simulink model "nonlinearpartd"  (R2017a)
settings: Solver=VariableStepAuto  StartTime=0.0  StopTime=3000  RelTol=1e-3
values from neighbouring files (symbols this model uses):
  g = 9.8    [CodeControlProject2.m]    (also in linear_system.m = 9.81; main.m; nonlinear_system.m = 9.81)
  Kc = lqr(A,B,Q,R)    [CodeControlProject2.m]
  l1 = 20    [CodeControlProject2.m]
  l2 = 10    [CodeControlProject2.m]
  M = 1000    [CodeControlProject2.m]    (also in main.m)
  m1 = 100    [CodeControlProject2.m]
  m2 = 100    [CodeControlProject2.m]
settings Model: Creator=Parth Jindal  LastModifiedBy=Parth Jindal

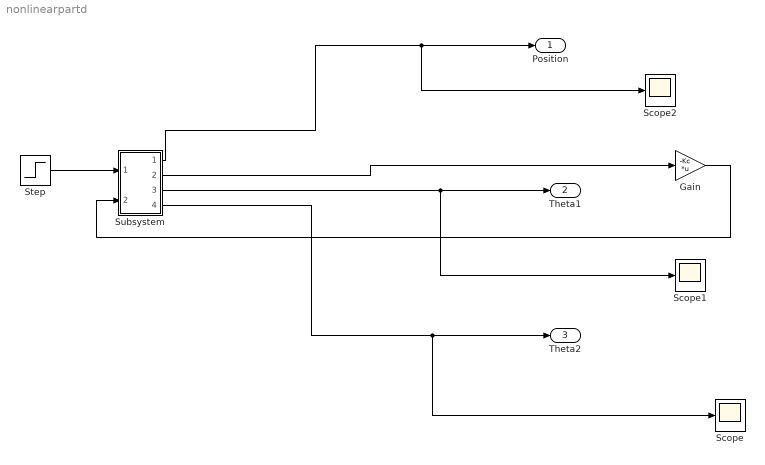
== system nonlinearpartd ==
  Gain : Gain  Gain=-Kc  Multiplication=Matrix(K*u)
  Scope : Scope
  Scope1 : Scope
  Scope2 : Scope
  Step : Step  SampleTime=0
  Subsystem : Subsystem
  Position : Outport
  Theta1 : Outport  Port=2
  Theta2 : Outport  Port=3
  wires:
  Subsystem/3(Out3) -> Scope1/1, Theta1/1
  Subsystem/4(Out4) -> Scope/1, Theta2/1
  Gain/1 -> Subsystem/2(In2)
  Subsystem/2(Out2) -> Gain/1
  Step/1 -> Subsystem/1(In1)
  Subsystem/1(Out1) -> Scope2/1, Position/1

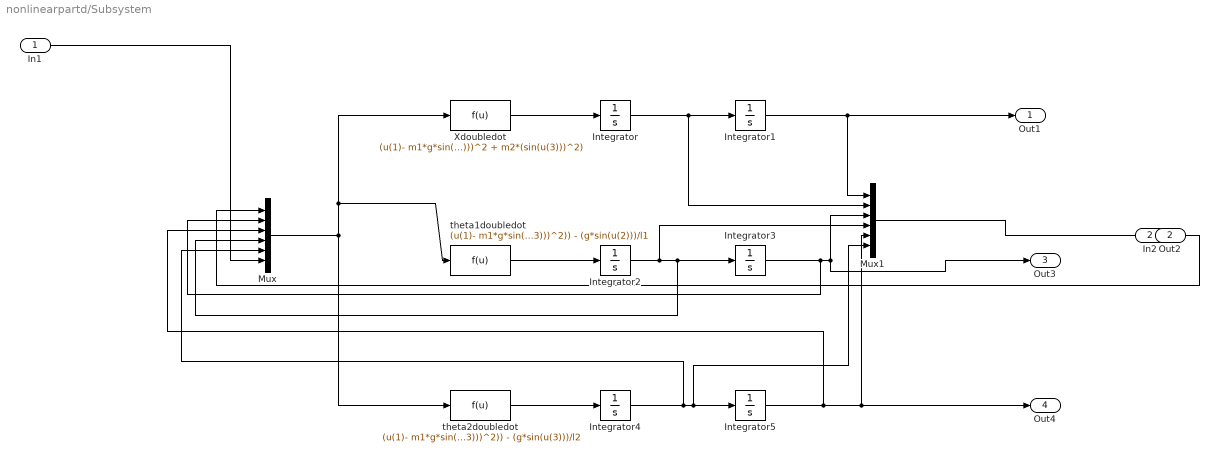
== system nonlinearpartd/Subsystem ==
  In1 : Inport
  In2 : Inport  Port=2
  Integrator{,2..5} (5 alike) : Integrator
  Integrator1 : Integrator  InitialCondition=-4
  Mux : Mux  Inputs=6
  Mux1 : Mux  Inputs=6
  Xdoubledot : Fcn  Expr=(u(1)- m1*g*sin(u(2))*cos(u(2)) - m1*l1*sin(u(2))*(u(4))^2 - m2*g*sin(u(3))*cos(u(3)) - m2*l2*sin(u(3))*(u(5))^2)/(M + m1*(sin(u(2)))^2 + m2*(sin(u(3)))^2)
  theta1doubledot : Fcn  Expr=(u(1)- m1*g*sin(u(2))*cos(u(2)) - m1*l1*sin(u(2))*(u(4))^2 - m2*g*sin(u(3))*cos(u(3)) - m2*l2*sin(u(3))*(u(5))^2)*cos(u(2))/(l1*(M + m1*(sin(u(2)))^2 + m2*(sin(u(3)))^2)) - (g*sin(u(2)))/l1
  theta2doubledot : Fcn  Expr=(u(1)- m1*g*sin(u(2))*cos(u(2)) - m1*l1*sin(u(2))*(u(4))^2 - m2*g*sin(u(3))*cos(u(3)) - m2*l2*sin(u(3))*(u(5))^2)*cos(u(3))/(l2*(M + m1*(sin(u(2)))^2 + m2*(sin(u(3)))^2)) - (g*sin(u(3)))/l2
  Out1 : Outport
  Out2 : Outport  Port=2
  Out3 : Outport  Port=3
  Out4 : Outport  Port=4
  wires:
  Integrator1/1 -> Out1/1, Mux1/1
  In1/1 -> Mux/6
  Integrator4/1 -> Mux/5, Mux1/6, Integrator5/1
  theta1doubledot/1 -> Integrator2/1
  Integrator5/1 -> Out4/1, Mux1/5, Mux/3
  In2/1 -> Mux/1
  theta2doubledot/1 -> Integrator4/1
  Mux/1 -> theta1doubledot/1, Xdoubledot/1, theta2doubledot/1
  Integrator2/1 -> Mux1/4, Mux/4, Integrator3/1
  Integrator3/1 -> Out3/1, Mux1/3, Mux/2
  Mux1/1 -> Out2/1
  Xdoubledot/1 -> Integrator/1
  Integrator/1 -> Mux1/2, Integrator1/1
